simulink model "simulink_model"  (R2023b)
settings: Solver=VariableStepAuto  StartTime=0.0  StopTime=10.0  RelTol=1e-3
settings Model: Creator=jbsantos  LastModifiedBy=jbsantos

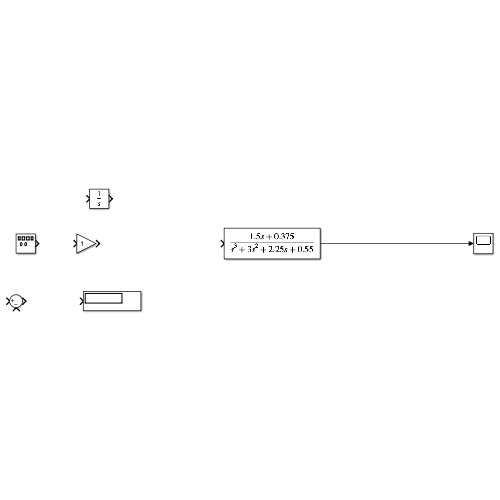
[thumbnail: Simulink's stored preview of the top-level diagram]
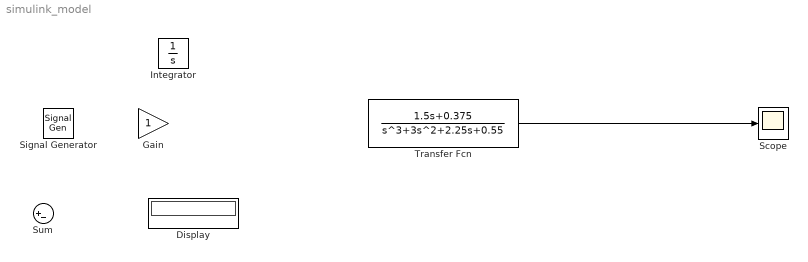
== system simulink_model ==
  Display : Display
  Gain : Gain
  Integrator : Integrator
  Scope : Scope
  Signal Generator : SignalGenerator  Units=rad/sec
  Sum : Sum  Inputs=|+-
  Transfer Fcn : TransferFcn  Numerator=[1.5 0.375]  Denominator=[1 3 2.25 0.55]
  wires:
  Transfer Fcn/1 -> Scope/1
